simulink model "Design_project_pid_audi_nonlinear"  (R2018a)
settings: Solver=VariableStepAuto  StartTime=0.0  StopTime=120  RelTol=1e-3
libraries: simulink x2
settings Model: Creator=DELL  LastModifiedBy=DELL

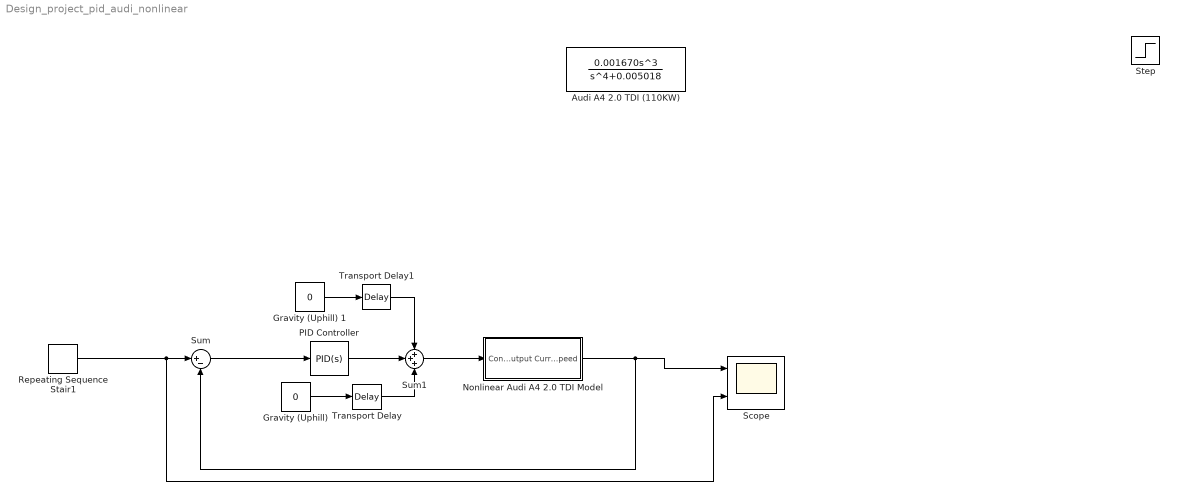
== system Design_project_pid_audi_nonlinear ==
  "Audi A4 2.0 TDI (110KW) " : TransferFcn  Numerator=[0.001670 0 0 0]  Denominator=[1 0 0 0 0.005018]
  "Gravity (Uphill) " : Constant  Value=0
  Gravity (Uphill) 1 : Constant  Value=0
  "Nonlinear Audi A4 2.0 TDI Model " : Subsystem
  PID Controller : simulink/Continuous/PID Controller  Controller=PID  TimeDomain=Continuous-time  SampleTime=-1  IntegratorMethod=Forward Euler  FilterMethod=Forward Euler  Form=Parallel  UseFilter=on  ControllerParametersSource=internal  P=147  I=1  D=3  N=100  InitialConditionSource=internal  InitialConditionForIntegrator=0  InitialConditionForFilter=0  ExternalReset=none  LimitOutput=off  UpperSaturationLimit=inf  LowerSaturationLimit=-inf  LinearizeAsGain=on  AntiWindupMode=none  Kb=1  TrackingMode=off  Kt=1  PParamMin=[]  PParamMax=[]  IParamMin=[]  IParamMax=[]  DParamMin=[]  DParamMax=[]  NParamMin=[]  NParamMax=[]  KbParamMin=[]  KbParamMax=[]  KtParamMin=[]  KtParamMax=[]  POutMin=[]  POutMax=[]  IOutMin=[]  IOutMax=[]  DOutMin=[]  DOutMax=[]  NOutMin=[]  NOutMax=[]  KbOutMin=[]  KbOutMax=[]  KtOutMin=[]  KtOutMax=[]  IntegratorOutMin=[]  IntegratorOutMax=[]  FilterOutMin=[]  FilterOutMax=[]  SumOutMin=[]  SumOutMax=[]  SumI1OutMin=[]  SumI1OutMax=[]  SumI2OutMin=[]  SumI2OutMax=[]  SumI3OutMin=[]  SumI3OutMax=[]  SumDOutMin=[]  SumDOutMax=[]  SaturationOutMin=[]  SaturationOutMax=[]  IntegratorContinuousStateAttributes=''  IntegratorStateMustResolveToSignalObject=off  IntegratorRTWStateStorageClass=Auto  FilterContinuousStateAttributes=''  FilterStateMustResolveToSignalObject=off  FilterRTWStateStorageClass=Auto  DifferentiatorICPrevScaledInput=0  DifferentiatorOutMin=[]  DifferentiatorOutMax=[]  FilterDiffOutCoefMin=[]  FilterDiffOutCoefMax=[]  SumDenOutMin=[]  SumDenOutMax=[]  SumNumOutMin=[]  SumNumOutMax=[]  ReciprocalOutMin=[]  ReciprocalOutMax=[]  DivideOutMin=[]  DivideOutMax=[]  TunerSelectOption=Transfer Function Based (PID Tuner App)
  Repeating Sequence Stair1 : simulink/Sources/Repeating Sequence Stair  OutValues=[10 20 40 80 110 90 60 30 10]  tsamp=8  OutMin=[]  OutMax=[]  OutDataTypeStr=int8  OutputDataTypeScalingMode=int8  OutDataType=fixdt(0,8)  ConRadixGroup=Best Precision: Vector-wise  OutScaling=2^-12
  Scope : Scope  NumInputPorts=2
  Step : Step  Time=0  After=100  SampleTime=0
  Sum : Sum  Inputs=|+-
  Sum1 : Sum  Inputs=+++
  Transport Delay : TransportDelay  DelayTime=24
  Transport Delay1 : TransportDelay  DelayTime=48
  wires:
  Sum/1 -> PID Controller/1
  Repeating Sequence Stair1/1 -> Scope/2, Sum/1
  "Gravity (Uphill) "/1 -> Transport Delay/1
  "Nonlinear Audi A4 2.0 TDI Model "/1(Current Speed) -> Sum/2, Scope/1
  PID Controller/1 -> Sum1/2
  Transport Delay/1 -> Sum1/3
  Transport Delay1/1 -> Sum1/1
  Gravity (Uphill) 1/1 -> Transport Delay1/1
  Sum1/1 -> "Nonlinear Audi A4 2.0 TDI Model "/1(Controller Output)

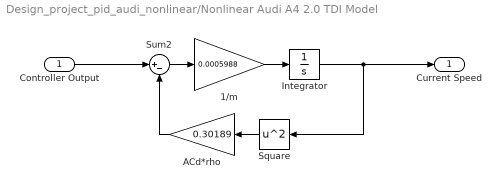
== system Design_project_pid_audi_nonlinear/Nonlinear Audi A4 2.0 TDI Model  ==
  Controller Output : Inport
  "1/m " : Gain  Gain=0.0005988
  ACd*rho : Gain  Gain=0.30189
  Integrator : Integrator
  Square : Math  Operator=square  SaturateOnIntegerOverflow=on
  Sum2 : Sum  Inputs=|+-
  Current Speed : Outport
  wires:
  ACd*rho/1 -> Sum2/2
  "1/m "/1 -> Integrator/1
  Sum2/1 -> "1/m "/1
  Integrator/1 -> Square/1, Current Speed/1
  Controller Output/1 -> Sum2/1
  Square/1 -> ACd*rho/1
